simulink model "Model4"  (R2022b)
settings: Solver=VariableStepAuto  StartTime=0.0  StopTime=inf  MaxStep=1e-3  RelTol=1e-3
model workspace (MAT data in the model file):
  Freq = Simulink.Parameter
  Freq.Value = 2000
  Freq.DataType = 'auto'
  Freq.Complexity = 'real'
  Freq.Dimensions = [1 1]
libraries: dspfdesign x2, commdigbbndam3 x2, commrandsrc3 x1
settings Model: Creator=Ceribro  LastModifiedBy=Ceribro

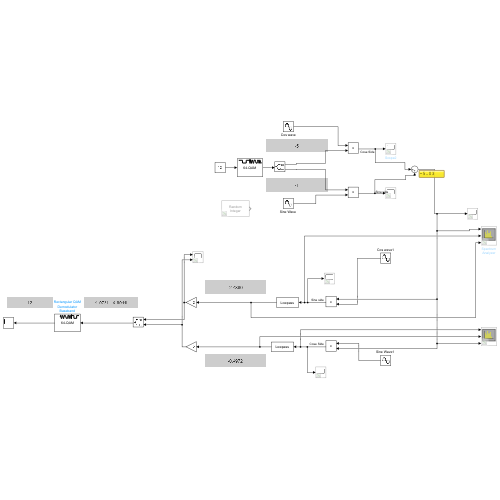
[thumbnail: Simulink's stored preview of the top-level diagram]
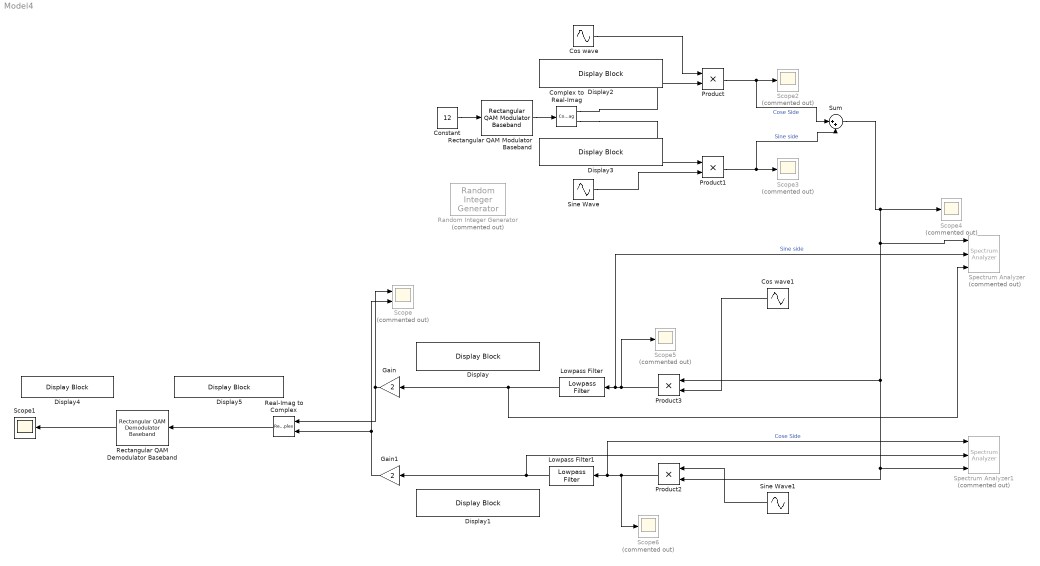
== system Model4 ==
  Complex to Real-Imag : ComplexToRealImag
  Constant : Constant  Value=12  SampleTime=0.01
  Cos wave : Sin  Frequency=2*pi*Freq  Phase=pi/2  SampleTime=1/44100  VectorParams1D=off
  Cos wave1 : Sin  Frequency=2*pi*Freq  Phase=pi/2  SampleTime=1/44100  VectorParams1D=off
  Display{,1..5} (6 alike) : DisplayBlock  LabelPosition=Hide  Transparency=1
  Gain : Gain  Gain=2
  Gain1 : Gain  Gain=2
  Lowpass Filter : dspfdesign/Lowpass Filter  FilterType=FIR  DesignForMinimumOrder=on  FilterOrder=50  PassbandFrequency=0.5e3  StopbandFrequency=1e3  PassbandRipple=0.1  StopbandAttenuation=80  InheritSampleRate=off  SampleRate=44100  SimulateUsing=Interpreted execution  roundingMode=Floor  coeffsDataTypeStr=fixdt(1,16)
  Lowpass Filter1 : dspfdesign/Lowpass Filter  FilterType=FIR  DesignForMinimumOrder=on  FilterOrder=50  PassbandFrequency=0.5e3  StopbandFrequency=1e3  PassbandRipple=0.1  StopbandAttenuation=80  InheritSampleRate=off  SampleRate=44100  SimulateUsing=Interpreted execution  roundingMode=Floor  coeffsDataTypeStr=fixdt(1,16)
  Product{,1..3} (4 alike) : Product
  Random Integer Generator : commrandsrc3/Random Integer Generator  Commented=on  SetSize=256  SeedSource=Auto  Seed=0  SampleTime=0.1  SamplesPerFrame=1  OutputDataType=double  SimulateUsing=Interpreted execution
  Real-Imag to Complex : RealImagToComplex
  Rectangular QAM Demodulator Baseband : commdigbbndam3/Rectangular QAM Demodulator Baseband  M=64  OutType=Integer  DecType=Hard decision  VarSource=Dialog  Variance=1  Dec=Binary  Mapping=[0:15]  PowType=Min. distance between symbols  MinDist=2  AvgPow=1  PeakPow=1  Ph=0  outDtype1=Inherit via internal rule  outDtype2=Inherit via internal rule  derotateFactorWordLen=16  derotateFactorDataTypeStr=Inherit: Same word length as input  derotateFactorLastDataTypeStr=Inherit: Same word length as input  denormFactorWordLen=16  denormFactorDataTypeStr=Inherit: Same word length as input  denormFactorLastDataTypeStr=Inherit: Same word length as input  prodOutWordLen=32  prodOutOverflowMode=Wrap  prodOutRoundingMode=Floor  prodOutOvFlMode=off  prodOutOvFlModeLastStrValue=off  sumWordLen=32
      settings: LibrarySourceBlock=|
      | commhdldigbbndam/Rectangular QAM
      | Demodulator
      | Baseband
  Rectangular QAM Modulator Baseband : commdigbbndam3/Rectangular QAM Modulator Baseband  M=64  InType=Integer  Enc=Binary  Mapping=[0:15]  PowType=Min. distance between symbols  MinDist=2  AvgPow=1  PeakPow=1  Ph=0  outDtype=Fixed-point  outWordLen=16  outUDDataType=sfix(16)  outFracLenMode=User-defined  outFracLen=0  outDataTypeStr=fixdt(1,16,0)  outLastDataTypeStr=fixdt(1,16,0)
      settings: LibrarySourceBlock=|
      | commhdldigbbndam/Rectangular QAM
      | Modulator
      | Baseband
  Scope : Scope  Commented=on  NumInputPorts=2
  Scope1 : Scope
  Scope{2..6} (5 alike) : Scope  Commented=on
  "Sine Wave " : Sin  Frequency=2*pi*Freq  SampleTime=1/44100  VectorParams1D=off
  "Sine Wave1 " : Sin  Frequency=2*pi*Freq  SampleTime=1/44100
  Spectrum Analyzer : SpectrumAnalyzer  Commented=on  NumInputPorts=3
  Spectrum Analyzer1 : SpectrumAnalyzer  Commented=on  NumInputPorts=3
  Sum : Sum  Inputs=|++
  wires:
  Rectangular QAM Modulator Baseband/1 -> Complex to Real-Imag/1
  Complex to Real-Imag/1 -> Product/2
  Complex to Real-Imag/2 -> Product1/1
  Product/1 -> Scope2/1, Sum/1  "Cose Side"
  Product1/1 -> Scope3/1, Sum/2  "Sine side"
  Sum/1 -> Spectrum Analyzer1/3, Product2/2, Product3/1, Spectrum Analyzer/1, Scope4/1
  Constant/1 -> Rectangular QAM Modulator Baseband/1
  Product3/1 -> Lowpass Filter/1, Spectrum Analyzer/2, Scope5/1  "Sine side"
  Product2/1 -> Spectrum Analyzer1/1, Lowpass Filter1/1, Scope6/1  "Cose Side"
  Lowpass Filter/1 -> Gain/1, Spectrum Analyzer/3
  Lowpass Filter1/1 -> Spectrum Analyzer1/2, Gain1/1
  Cos wave1/1 -> Product3/2
  "Sine Wave1 "/1 -> Product2/1
  "Sine Wave "/1 -> Product1/2
  Cos wave/1 -> Product/1
  Gain/1 -> Scope/1, Real-Imag to Complex/1
  Gain1/1 -> Real-Imag to Complex/2, Scope/2
  Real-Imag to Complex/1 -> Rectangular QAM Demodulator Baseband/1
  Rectangular QAM Demodulator Baseband/1 -> Scope1/1
